simulink model "temp_mmms4th"  (R2024b)
settings: Solver=VariableStepAuto  StartTime=0.0  StopTime=10.0  RelTol=1e-3
values from neighbouring files (symbols this model uses):
  iota0 = eye(6,6)    [Initiate_KUKA_inv.m]    (also in Main_MMMS.m; test_KUKA_elements.m)
  K_d = 10*[1.3*eye(3) zeros(3);zeros(3) 0.8*eye(3)]    [Initiate_FQ.m]    (also in Initiate_KUKA_inv.m = 5*[0.7*eye(3) zeros(3);zeros(3) 0.5*eye(3)]; MMMS_Initiate_FQ.m; Main_MMMS.m = 5*[0.7*eye(3) zeros(3);zeros(3) 0.5*eye(3)]; test_KUKA_elements.m = 50*[0.7*eye(3) zeros(3);zeros(3) 0.5*eye(3)])
  K_i = 5*[0.1*eye(3) zeros(3);zeros(3) 0.01*eye(3)]    [Initiate_FQ.m]    (also in Initiate_KUKA_inv.m = 5*[0.01*eye(3) zeros(3);zeros(3) 0.001*eye(3)]; MMMS_Initiate_FQ.m; Main_MMMS.m = 5*[0.01*eye(3) zeros(3);zeros(3) 0.001*eye(3)]; test_KUKA_elements.m = 50*[0.01*eye(3) zeros(3);zeros(3) 0.001*eye(3)])
  K_p = 100*[0.1 0 0 0 0 0;0 0.1 0 0 0 0; 0 0 0.1 0 0 0; 0 0 0 0.01 0 0 ... (first row only)    [Initiate_FQ.m]    (also in Initiate_KUKA_inv.m = 5*[0.1 0 0 0 0 0;0 0.1 0 0 0 0; 0 0 0.1 0 0 0; 0 0 0 0.01 0 ; MMMS_Initiate_FQ.m; Main_MMMS.m = 5*[0.1 0 0 0 0 0;0 0.1 0 0 0 0; 0 0 0.1 0 0 0; 0 0 0 0.01 0 ; test_KUKA_elements.m = 50*[0.1 0 0 0 0 0;0 0.1 0 0 0 0; 0 0 0.1 0 0 0; 0 0 0 0.01 0)
  K_w = 200*eye(7)    [Initiate_FQ.m]    (also in MMMS_Initiate_FQ.m)
  K_wd = 2*eye(7)    [Initiate_FQ.m]    (also in MMMS_Initiate_FQ.m)
  M0 = M_temp.M0.data(:,:,1)    [Initiate_FQ.m]    (also in MMMS_Initiate_FQ.m; test_KUKA_elements.m)
  m0_frak = diag_M(1:6,1:6)    [Initiate_KUKA_inv.m]    (also in Main_MMMS.m; make_uncertain.m = diag_M_unc(1:6,1:6); test_KUKA_elements.m)
  M0m = M_temp.M0m.data(:,:,1)    [Initiate_FQ.m]    (also in MMMS_Initiate_FQ.m; test_KUKA_elements.m)
  m_diag = diag_M(7:end,7:end)    [Initiate_KUKA_inv.m]    (also in Main_MMMS.m; make_uncertain.m = diag_M_unc(7:end,7:end); test_KUKA_elements.m)
  M_t = (((Adjoint(g_It))'\M_t_body)/(Adjoint(g_It)))    [Initiate_FQ.m]    (also in Initiate_KUKA_inv.m = [eye(3)*mt zeros(3); zeros(3) eye(3)*80]; MMMS_Initiate_FQ.m; Main_MMMS.m = [eye(3)*mt zeros(3); zeros(3) eye(3)*80]; test_KUKA_elements.m = [eye(3)*mt zeros(3); zeros(3) eye(3)*80])
  M_t_body = [eye(3)*mt zeros(3); zeros(3) eye(3)*0.416667]    [Initiate_FQ.m]    (also in MMMS_Initiate_FQ.m)
  mu = P0    [Initiate_FQ.m]    (also in Initiate_KUKA_inv.m = zeros(6,1); MMMS_Initiate_FQ.m; Main_MMMS.m = zeros(6,1); make_uncertain.m = P0_unc)
  mu_t = inv((Adjoint(g_It))')*M_t_body*[V_It;w_t]    [Initiate_FQ.m]    (also in Initiate_KUKA_inv.m = M_t*[V_0t;w_t]; MMMS_Initiate_FQ.m; Main_MMMS.m = M_t*[V_0t;w_t]; make_uncertain.m = inv((Adjoint(g_It))')*M_t_body_unc*[V_It;w_t])
  sc_size = 1    [Initiate_KUKA_inv.m]    (also in Main_MMMS.m; test_KUKA_elements.m)
  Xi_m_matrix = zeros(6*n,n)    [Initiate_KUKA_inv.m]    (also in Main_MMMS.m)
undefined symbols (not defined in the file or in its folder): Mm, Xi_m
(part 2 of 2)

== matlab function temp_mmms4th/Feedback Transformation3/Inverse Dynamics1/C_hat1/Lm_partials1/Lm0partial_par ==
  data: q_m input; Lm0_partial_par output; Xi_m input; iota0 input
function Lm0_partial_par = Lm0_partial_par(q_m,Xi_m,iota0)
% Calculates the C_hat_m matrix from base pose and arm joint angles

n=length(q_m);

% Find partial of Lm to joint angles
Lm0_partial_par=zeros(6*n,6,n,n); % 6nx6xn
for i=1:n
    for k=1:n
        for j=1:n
            Lm0_partial_par(6*(j-1)+1:6*j,1:6,i,k)=Ad_partial_par(j,1,i,k,Xi_m,q_m,iota0); % equation 114 of TRO paper
        end
    end
end

%%%%%%%%%%%%%%%%%%%%%%%%%%%%%%%%%%%%%%%%%%%%%%%%%%%%%%%%%%%%% MUST BE
%%%%%%%%%%%%%%%%%%%%%%%%%%%%%%%%%%%%%%%%%%%%%%%%%%%%%%%%%%%%% CHECKED


% Lm0_partial_par

== matlab function temp_mmms4th/Feedback Transformation3/Inverse Dynamics1/C_hat1/Lm_partials1/Lmpartial ==
  data: q_m input; Lm_partial output; Xi_m input; iota0 input
function Lm_partial  = Lm_partial(q_m,Xi_m,iota0)
% Calculates the C_hat_m matrix from base pose and arm joint angles

n=length(q_m);

% Find partial of Lm0 to joint angles
Lm_partial=zeros(6*n,6*n,n); % 6nx6xn
for i=1:n
    Lm_partial(:,:,i)=zeros(6*n,6*n);
    for j=2:n
        for k=2:n
            if j>i && i>=k
                Lm_partial(6*(j-1)+1:6*j,6*(k-2)+1:6*(k-1),i)=Ad_partial(j,k,i,Xi_m,q_m,iota0); % equation 81 of TRO paper
            elseif i==j && i>=k
                Lm_partial(6*(j-1)+1:6*j,6*(k-2)+1:6*(k-1),i)=Ad_partial(j,k,i,Xi_m,q_m,iota0); % equation 81 of TRO paper
            else
                Lm_partial(6*(j-1)+1:6*(j-1)+6,6*(k-2)+1:6*(k-2)+6,i)=zeros(6,6);
            end

        end
    end
end

== matlab function temp_mmms4th/Feedback Transformation3/Inverse Dynamics1/C_hat1/Lm_partials1/Lmpartial_par ==
  data: q_m input; Lm_partial_par output; Xi_m input; iota0 input
function Lm_partial_par  = Lm_partial_par(q_m,Xi_m,iota0)
% Calculates the C_hat_m matrix from base pose and arm joint angles

n=length(q_m);

% Find partial of Lm0 to joint angles
Lm_partial_par=zeros(6*n,6*n,n,n); % 6nx6xn
for i=1:n
    for s=1:n
        Lm_partial_par(:,:,i,s)=zeros(6*n,6*n);
        for j=2:n
            for k=2:n
                if j>i && i>=k
                    Lm_partial_par(6*(j-1)+1:6*j,6*(k-2)+1:6*(k-1),i,s)=Ad_partial_par(j,k,i,s,Xi_m,q_m,iota0); % equation 81 of TRO paper
                elseif i==j && i>=k
                    Lm_partial_par(6*(j-1)+1:6*j,6*(k-2)+1:6*(k-1),i,s)=Ad_partial_par(j,k,i,s,Xi_m,q_m,iota0); % equation 81 of TRO paper
                else
                    Lm_partial_par(6*(j-1)+1:6*(j-1)+6,6*(k-2)+1:6*(k-2)+6,i,s)=zeros(6,6);
                end
            end
        end
    end
end

% Lm_partial_par

== matlab function temp_mmms4th/Feedback Transformation3/Inverse Dynamics1/C_hat1/M_partials1/ M0partial ==
  data: q_m input; M0_partial output; Lm0 input; V input; iota0 input; diag_Mm input; Lm0_partial input
function M0_partial = M0_partial(q_m,Lm0,V,iota0,diag_Mm,Lm0_partial)
% Calculates the C_hat_m matrix from base pose and arm joint angles

n=length(q_m);
b=length(V);

% Find partial of M0 to joint angles
M0_partial=zeros(b,b,n); %initiate
for i=1:n
    temp1=transpose(Lm0_partial(1:end,1:end,i))*diag_Mm*Lm0;
    temp2=transpose(Lm0)*diag_Mm*Lm0_partial(1:end,1:end,i);
    M0_partial(1:b,1:b,i)= iota0'*(temp1+temp2)*iota0; %6x6 %equation 117 of TRO
end

== matlab function temp_mmms4th/Feedback Transformation3/Inverse Dynamics1/C_hat1/M_partials1/ M0partial_par ==
  data: q_m input; M0_partial_par output; Lm0 input; V input; iota0 input; diag_Mm input; Lm0_partial input; Lm0_partial_par input
function M0_partial_par = M0_partial_par(q_m,Lm0,V,iota0,diag_Mm,Lm0_partial,Lm0_partial_par)
% Calculates the C_hat_m matrix from base pose and arm joint angles

n=length(q_m);
b=length(V);

% Find partial of M0 to joint angles
M0_partial_par=zeros(b,b,n,n); %initiate
for i=1:n
    for s=1:n
        temp1=(Lm0_partial_par(1:end,1:end,i,s))'*diag_Mm*Lm0;
        temp2=(Lm0_partial(1:end,1:end,i))'*diag_Mm*Lm0_partial(1:end,1:end,s);
        temp3=(Lm0_partial(1:end,1:end,s))'*diag_Mm*Lm0_partial(1:end,1:end,i);
        temp4=(Lm0)'*diag_Mm*Lm0_partial_par(1:end,1:end,i,s);
        M0_partial_par(1:b,1:b,i,s)= iota0'*(temp1+temp2+temp3+temp4)*iota0; %6x6 %equation 117 of TRO
    end
end

% M0_partial_par

== matlab function temp_mmms4th/Feedback Transformation3/Inverse Dynamics1/C_hat1/M_partials1/M0mpartial ==
  data: q_m input; M0m_partial output; V input; Lm input; Lm0 input; iota0 input; diag_Mm input; Lm0_partial input; Lm_partial input; Xi_m_matrix input
function M0m_partial = M0m_partial(q_m,V,Lm,Lm0,iota0,diag_Mm,Lm0_partial,Lm_partial, Xi_m_matrix)
% Calculates the C_hat_m matrix from base pose and arm joint angles

n=length(q_m);
b=length(V);

% Find partial of M0m to joint angles
M0m_partial=zeros(b,n,n);
for i=1:n
    temp1=transpose(Lm0_partial(1:end,1:end,i))*diag_Mm*Lm;
    temp2=transpose(Lm0)*diag_Mm*Lm_partial(1:end,1:end,i);
    M0m_partial(1:b,1:n,i)= iota0'*(temp1+temp2)*Xi_m_matrix; % equation 118 of TRO paper
end

== matlab function temp_mmms4th/Feedback Transformation3/Inverse Dynamics1/C_hat1/M_partials1/M0mpartial_par ==
  data: q_m input; M0m_partial_par output; V input; Lm input; Lm0 input; iota0 input; diag_Mm input; Lm0_partial input; Lm_partial input; Xi_m_matrix input; Lm0_partial_par input; Lm_partial_par input
function M0m_partial_par = M0m_partial_par(q_m,V,Lm,Lm0,iota0,diag_Mm,Lm0_partial,Lm_partial, Xi_m_matrix,Lm0_partial_par,Lm_partial_par)
% Calculates the C_hat_m matrix from base pose and arm joint angles

n=length(q_m);
b=length(V);

% Find partial of M0m to joint angles
M0m_partial_par=zeros(b,n,n,n);
for i=1:n
    for s=1:n
        temp1=transpose(Lm0_partial_par(1:end,1:end,i,s))*diag_Mm*Lm;
        temp2=transpose(Lm0_partial(1:end,1:end,i))*diag_Mm*Lm_partial(1:end,1:end,s);
        temp3=transpose(Lm0_partial(1:end,1:end,s))*diag_Mm*Lm_partial(1:end,1:end,i);
        temp4=transpose(Lm0)*diag_Mm*Lm_partial_par(1:end,1:end,i,s);
        M0m_partial_par(1:b,1:n,i,s)= iota0'*(temp1+temp2+temp3+temp4)*Xi_m_matrix; % equation 118 of TRO paper
    end
end


% M0m_partial_par

== matlab function temp_mmms4th/Feedback Transformation3/Inverse Dynamics1/C_hat1/M_partials1/Mmpartial ==
  data: q_m input; Mm_partial output; Xi_m_matrix input; Lm input; diag_Mm input; Lm_partial input
function Mm_partial = Mm_partial(q_m,Xi_m_matrix,Lm,diag_Mm,Lm_partial)
% Calculates the C_hat_m matrix from base pose and arm joint angles

n=length(q_m);

% find the non-generalized arm mass matrix'x derivative to joint angles
Mm_partial=zeros(n,n,n);
for i=1:n
    temp=   transpose(Lm_partial(1:6*n,1:6*n,i))*diag_Mm*Lm  +   transpose(Lm)*diag_Mm*Lm_partial(1:6*n,1:6*n,i);
    Mm_partial(1:n,1:n,i)=transpose(Xi_m_matrix)*temp*Xi_m_matrix; %calcualte the derivative of not-augmented arm mass matrix from equation 120 of TRO paper
end

== matlab function temp_mmms4th/Feedback Transformation3/Inverse Dynamics1/C_hat1/Mm_hat_partial1 ==
  data: q_m input; AMA_partial input; Mm_hat_partial output; Mm_partial input
function Mm_hat_partial = Mm_hat_partial(q_m, AMA_partial, Mm_partial)
% Calculates the C_hat_m matrix from base pose and arm joint angles

n=length(q_m);

% find the generalized arm mass matrix'x derivative to joint angles
Mm_hat_partial=zeros(n,n,n);
for i=1:n
    Mm_hat_partial(1:n,1:n,i)=Mm_partial(1:n,1:n,i)-AMA_partial(1:n,1:n,i); %calcualte the derivative of augmented arm mass matrix from equation 119 of TRO paper
end

== matlab function temp_mmms4th/Feedback Transformation3/Inverse Dynamics1/Inverse Dynamics/Ad_g_I0_dot ==
  data: g_I0 input; V_I0 input; Ad_g_I0_dot output
function Ad_g_I0_dot = Ad_g_I0_dot(g_I0,V_I0)
% Calculation of F_mu Eq 30 of paper
Ad_g_I0_dot=adjoint_low(V_I0)'*Adjoint(g_I0)';
% adjoint_low(V_I0)*transpose(Adjoint*(g_I0)))

== matlab function temp_mmms4th/Feedback Transformation3/Inverse Dynamics1/Inverse Dynamics/Ad_g_I0_dot1 ==
  data: V_t input; Ad_g_It_dot output; g_It input
function Ad_g_It_dot = Ad_g_It_dot(V_t,g_It)
% Calculation of F_mu Eq 30 of paper
Ad_g_It_dot=adjoint_low(V_t)'*Adjoint(g_It)';

== matlab function temp_mmms4th/Feedback Transformation3/Inverse Dynamics1/Inverse Dynamics/Ad_g_te_dot ==
  data: V_te input; Ad_g_te_dot output; g_te input
function Ad_g_te_dot = Ad_g_te_dot(V_te,g_te)
% Calculation of F_mu Eq 30 of paper
Ad_g_te_dot=-adjoint_low(V_te)/Adjoint(g_te);

== matlab function temp_mmms4th/Controller4/Hes w ==
  data: A input; Hes_w output; A_partial input; A_partial_par input; grad_w input; q_dot input
function Hes_w  = Hes_w(A,A_partial,A_partial_par,grad_w, q_dot)

w=sqrt(det(A*A'));

n=length(q_dot);
Hes_w=zeros(n,n);
for i=1:n
    for s=1:n
        AAT_partial_i=A*A_partial(:,:,i)'+A_partial(:,:,i)*A';
        AAT_partial_s=A*A_partial(:,:,s)'+A_partial(:,:,s)*A';
        AAT_partial_is=A_partial(:,:,s)*A_partial(:,:,i)'+A_partial(:,:,i)*A_partial(:,:,s)'+A*A_partial_par(:,:,i,s)'+A_partial_par(:,:,i,s)*A';
        temp1=(A*A')\AAT_partial_s;
        temp2 = (A*A')\AAT_partial_i;

        Hes_w(i,s) = 0.5*grad_w(s)* trace( temp2) + (w/2)*trace(-temp1*temp2+(A*A')\AAT_partial_is);%det(A*A')*trace(inv(A')A_dot'+inv(A')*inv(A)*A_dot*A');
    end
end

% w_dot=1/norm(grad_w'*q_dot);

== matlab function temp_mmms4th/Feedback Transformation3/Inverse Dynamics1/Inverse Dynamics/FU ==
  data: MmJcross input; F_U output
function F_U = F_U(MmJcross)
F_U=MmJcross;

== matlab function temp_mmms4th/Feedback Transformation3/Inverse Dynamics1/Inverse Dynamics/Fm ==
  data: MmJcross input; F_m output; A_dot input; Cm_hat input
function F_m = F_m(MmJcross,A_dot,Cm_hat)
% Calculation of F_mu Eq 30 of paper
F_m=MmJcross*(A_dot)+Cm_hat;

== matlab function temp_mmms4th/Feedback Transformation3/Inverse Dynamics1/Inverse Dynamics/Fmu ==
  data: MmJcross input; M0 input; M_0_dot input; g_I0 input; F_mu output; Ad_g_I0_dot input
function F_mu = F_mu(MmJcross,M0,M_0_dot,g_I0,Ad_g_I0_dot)
% Calculation of F_mu Eq 30 of paper
F_mu=-MmJcross*(M0\M_0_dot*inv(M0)*transpose(Adjoint(g_I0))+ ...
    M0\Ad_g_I0_dot);

== matlab function temp_mmms4th/Feedback Transformation3/Inverse Dynamics1/Inverse Dynamics/MATLAB Function3 ==
  data: MmJcross input; g_te input; F_t output; g_It input; Mt input; Ad_gte_dot input; Ad_gIt_dot input
function F_t = F_t(MmJcross,g_te,g_It,Mt,Ad_gte_dot,Ad_gIt_dot)
% Calculation of F_mu Eq 30 of paper
F_t=-MmJcross*(Ad_gte_dot/Mt*Adjoint(g_It)'+Adjoint(g_te)\(Mt\Ad_gIt_dot));

% F_t=MmJcross*(-adjoint_low(V_te)/Adjoint(g_te)/Adjoint(g_tt)/M_t/Adjoint(g_It)'+...
%     Adjoint()\); 

% J_e0_dot*inverse(M0)*transpose(Adjoint*(g_I0))- ...
%     J_e0*inverse(M0)*M_0_dot*inverse(M0)*transpose(Adjoint*(g_I0))+ ...
%     J_e0*inverse(M0)*adjoint_low(inverse(M0*transpose(Adjoint(g_I0))*mu)-A*q_dot_m)
%     Ad_g_te_dot

== matlab function temp_mmms4th/Feedback Transformation3/Inverse Dynamics1/Inverse Dynamics/MmJcross ==
  data: Mm_hat input; MmJcross output; A input
function MmJcross = MmJcross(Mm_hat, A)

JJ=-A;

A_dagger = ((Mm_hat)\JJ')/((JJ/Mm_hat)*JJ');
MmJcross = Mm_hat*A_dagger;%,10^(-2));

== matlab function temp_mmms4th/Feedback Transformation3/Inverse Dynamics1/Inverse Dynamics/Mm_hat ==
  data: M0 input; Mm_hat output; Mm input; A input
function Mm_hat = Mm_hat(M0,Mm,A)

Mm_hat=Mm-A'*M0*A;

== matlab function temp_mmms4th/Feedback Transformation3/Inverse Dynamics1/M0_dot ==
  data: M0_partial input; q_m_dot input; M0_dot output
function M0_dot = fcn(M0_partial, q_m_dot)
n=length(q_m_dot);

M0_dot=zeros(6,6);
for i=1:n
    M0_dot=M0_dot+M0_partial(:,:,i).*q_m_dot(i);
end

== matlab function temp_mmms4th/Feedback Transformation3/Inverse Dynamics1/N_hat/N_hat ==
  data: N_hat_temp output; q_m input; q_dot_m input; A input; V input; P input; M0_partial input; A_partial input; iota0 input; M0 input
function N_hat_temp = N_hat(q_m,q_dot_m,A,V,P,M0_partial, A_partial, iota0, M0)
% Calculates the N_hat_m matrix from base pose and arm joint angles

n=length(q_m);
b=length(V);

%Form N_hat from equation 19 of ACC paper
N_temp1=zeros(n,b); N_temp2=zeros(n,b); N_temp3=zeros(n,b);

for i=1:n
    N_temp1=N_temp1+transpose(squeeze(A_partial(1:b,1:n,i)).*q_dot_m(i)); % transpose of (bxn times 1x1) 
    N_temp2(i,1:b)=transpose(q_dot_m)*transpose(squeeze(A_partial(1:b,1:n,i))); %1xn times nxb
    N_temp3(i,1:b)=0.5*transpose(P)*(-M0\M0_partial(1:end,1:end,i)/M0); % 1xb times bxb
end

N_hat_temp=transpose(A)*transpose(adjoint_low(V,iota0))-N_temp1+N_temp2+N_temp3;

== matlab function temp_mmms4th/Feedback Transformation3/Inverse Dynamics1/N_hat1/MATLAB Function ==
  data: g_I0 input; V_Ie output; V_Ie_e input
function V_Ie = fcn(g_I0,V_Ie_e)

V_Ie = Adjoint(g_I0)\V_Ie_e;

== matlab function temp_mmms4th/Feedback Transformation3/Inverse Dynamics1/N_hat1/N_hat ==
  data: N_hat_temp output; q_m input; q_dot_m input; A input; V input; P input; M0_partial input; A_partial input; iota0 input; M0 input
function N_hat_temp = N_hat(q_m,q_dot_m,A,V,P,M0_partial, A_partial, iota0, M0)
% Calculates the N_hat_m matrix from base pose and arm joint angles

n=length(q_m);
b=length(V);

%Form N_hat from equation 19 of ACC paper
N_temp1=zeros(n,b); N_temp2=zeros(n,b); N_temp3=zeros(n,b);

for i=1:n
    N_temp1=N_temp1+transpose(squeeze(A_partial(1:b,1:n,i)).*q_dot_m(i)); % transpose of (bxn times 1x1) 
    N_temp2(i,1:b)=transpose(q_dot_m)*transpose(squeeze(A_partial(1:b,1:n,i))); %1xn times nxb
    N_temp3(i,1:b)=0.5*transpose(P)*(M0\squeeze(M0_partial(1:end,1:end,i)))/(M0); % 1xb times bxb
end

N_hat_temp=-transpose(A)*transpose(adjoint_low(V,iota0))-N_temp1+N_temp2+N_temp3;

== matlab function temp_mmms4th/Dynamic Parameters3/ 1 ==
  data: q_m input; L0 output; Lm0 output; Lm output; Xi_m input
function [L0,Lm0,Lm] =L_calculator(q_m,Xi_m)
% Calculates the time-dependent L matrix
n=length(q_m);
L=zeros(6*(n+1),6*(n+1));
% Compute M_frak for ith body
% Calculate L matrix
for i=1:n+1
    for j=1:n+1
        if i>j
            Ad_temp=eye(6);
            for k=j:i-1
                Ad_temp=Adjoint(g_Matrix(-Xi_m(:,k),q_m(k)))*Ad_temp;
            end
            L(6*(i-1)+1:6*(i-1)+6,6*(j-1)+1:6*(j-1)+6)=Ad_temp;
        elseif i==j
            L(6*(i-1)+1:6*(i-1)+6,6*(j-1)+1:6*(j-1)+6)=eye(6);
        elseif i<j
            L(6*(i-1)+1:6*(i-1)+6,6*(j-1)+1:6*(j-1)+6)=zeros(6);
        end
    end
end

L0=L(1:6,1:6);
Lm0=L(7:end,1:6);
Lm=L(7:end,7:end);

end

== matlab function temp_mmms4th/Controller4/Kinematics/MATLAB Function ==
  data: g_I0 input; V_Ie output; V_Ie_e input
function V_Ie = fcn(g_I0,V_Ie_e)

V_Ie = Adjoint(g_I0)*V_Ie_e;

== matlab function temp_mmms4th/Dynamic Parameters3/MATLAB Function ==
  data: A input; wt output
function wt = fcn(A)

J=-A;
% SVD=svd(J);

% minSVD=min(SVD);
% maxSVD=max(SVD);

wt=sqrt(det(J*J'));

% y = minSVD/maxSVD;

== matlab function temp_mmms4th/Dynamic Parameters3/MATLAB Function1 ==
  data: g_I0 input; mu input; P output
function P=Momentum(g_I0,mu)
% find the momentum in current base frame
P=Adjoint(g_I0)'*mu;

== matlab function temp_mmms4th/Dynamic Parameters3/V_I1 ==
  data: P input; A_connection input; q_dot_m input; M0 input; V_I0 output; g_I0 input
function V_I0 = V_I0(P, A_connection, q_dot_m, M0, g_I0)
V_I0=Adjoint(g_I0)*((M0\P)-A_connection*q_dot_m);

== matlab function temp_mmms4th/Controller4/Kinematics/Pose Error Function ==
  data: g_te input; E_g output
function E_g = pose_Error_function(g_te)
% Calculates the pose Error function from the relative pose of end-effector to target
R_te=g_te(1:3,1:3);
p_te=g_te(1:3,4);

temp_R=eye(3)-R_te;
temp_R=0.5*trace(temp_R);

temp_p=0.5*transpose(p_te)*p_te;
E_g =temp_R+temp_p;

== matlab function temp_mmms4th/Controller4/Kinematics/V_It_1 ==
  data: V_I0 input; g_I0 input; V_I0_3 output
function V_I0_3 = V_I03(V_I0, g_I0)


% g_gpt=[eye(3) [0.25; 0.25; 0.25]; 0 0 0 1];
R=g_I0(1:3,1:3);

V_I0_3=Adjoint(g_I0)*[R zeros(3);zeros(3) R]'*V_I0; %[R zeros(3);zeros(3) R]


% Ad g_Igp(t) M^-1 Ad gI_gp(t)' inv(Ad g_I_gp') Mt inv (Ad g_I_gp) V_Igp

== matlab function temp_mmms4th/Controller4/Kinematics/Velocity_error ==
  data: g_I0 input; V_Ie input; V_e output; V_It input; g_It input; normV output
function [V_e,normV] = Velocity_Error_function(g_I0, V_Ie,V_It, g_It)
% Calculates the Velocity Error function from the momentums of chaser and
% target and the joint velocities

Rt=g_It(1:3,1:3);
R0=g_I0(1:3,1:3);

V_te_I=V_Ie-V_It; %Adjoint(inv(g_I0))*
V_te=Adjoint(inv(g_I0))*V_te_I;
V_e=V_te;

normV=norm(V_e);

== matlab function temp_mmms4th/Controller4/Nullspace derivatives ==
  data: Mm input; A input; N_dot output; Mm_partial input; A_partial input; q_dot input; Z_dot output; j input; Nj input
function [N_dot,Z_dot] =Nullspace_derivatives(Mm,A,Mm_partial,A_partial,q_dot,j, Nj)

Mm_dot=zeros(7);
A_dot=zeros(6,7);
for i=1:length(Mm_partial(1,1,:))
    Mm_dot=Mm_dot+Mm_partial(:,:,i).*q_dot(i);
    A_dot=A_dot+A_partial(:,:,i).*q_dot(i);
end

%parts of N_dot

N1=((Mm\Mm_dot)/Mm)     *   A'   / ((A/Mm)*A')*A;
N2=-Mm\A_dot'   /   ((A/Mm)*A')   * A;
N3=(Mm\A')   /   ((A/Mm)*A')    * ((A_dot/Mm)*A'  -   (A/Mm) *(Mm_dot /Mm) *A'    +   (A/Mm)*A_dot') /   ((A/Mm)*A')   *   A;
N4=-(Mm\ A') *    ((A/Mm)*A')  *A_dot;

N_dot=N1+N2+N3+N4;

% Z_dot=N_dot(:,j);%/norm_Z;
Nj_dot=N_dot(:,j);

Z_dot=Nj_dot/norm(Nj)-Nj'*Nj_dot*Nj/norm(Nj)^3;
